simulink model "runner"  (Simulink 7.2)
settings: Solver=ode45  StartTime=0.0  StopTime=2  RelTol=1e-3
undefined symbols (not defined in the file or in its folder): controller_runner, drawRunner, P
libraries: simulink x1
settings Model: Creator=beard  LastModifiedBy=Andrew
settings OptimizationCC: InitFltsAndDblsToZero=on
settings DebuggingCC: StrictBusMsg=ErrorLevel1
settings CodeAppCC: CustomSymbolStrType=$N$R$M_T
settings GRTTargetCC: TargetFunctionLibrary=NOT IN USE  CPPClassGenCompliant=on

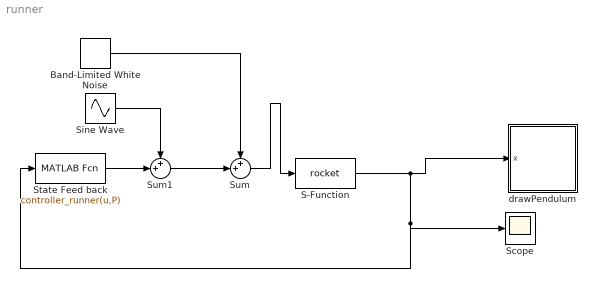
== system runner ==
  Band-Limited White Noise : simulink/Sources/Band-Limited White Noise  SystemSampleTime=-1  Cov=[0]  Ts=0.1  seed=[23341]
  S-Function : S-Function  FunctionName=rocket  Parameters=P  EnableBusSupport=off
  Scope : Scope
      settings: YMin=-12  YMax=1
  Sine Wave : Sin  Amplitude=0.1  Frequency=10  SampleTime=0
  State Feed back : MATLABFcn  MATLABFcn=controller_runner(u,P)  OutputDimensions=2
  Sum : Sum  Inputs=++|
  Sum1 : Sum  Inputs=++|
  drawPendulum : Subsystem
  wires:
  State Feed back/1 -> Sum1/2
  Sum1/1 -> Sum/2
  Sum/1 -> S-Function/1
  Band-Limited White Noise/1 -> Sum/1
  Sine Wave/1 -> Sum1/1
  S-Function/1 -> drawPendulum/1(x), Scope/1, State Feed back/1

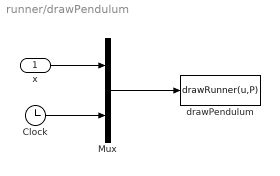
== system runner/drawPendulum ==
  x : Inport
  Clock : Clock
      settings: Decimation=10
  Mux : Mux  Inputs=2
  drawPendulum : MATLABFcn  MATLABFcn=drawRunner(u,P)  OutputDimensions=0  SampleTime=0.1
  wires:
  Mux/1 -> drawPendulum/1
  x/1 -> Mux/1
  Clock/1 -> Mux/2
